simulink model "Receiver"  (R2017b)
settings: Solver=FixedStepDiscrete  StartTime=0.0  StopTime=10.0  RelTol=1e-3
InitFcn:
  | modelSettings
undefined symbols (not defined in the file or in its folder): crcDecodeLag, numTrainingSamples, RadioSampleRate, VibertiTracebackLength, xPreambleSeq
libraries: dsphdlfiltering x19, simulink x7, hdlsllib x4, commdigbbndpm3 x2, commcrc2 x1, dspstat3 x1, commseqgen3 x1, commutil2 x1, commcnvcod2 x1
(part 1 of 2)
settings Model: DataTypeOverride=Off  MinMaxOverflowLogging=MinMaxAndOverflow  FPTRunName=NoOverride  Creator=tcollins  LastModifiedBy=tcollins
settings DataIOCC: SaveOutput=off  SaveTime=off
settings OptimizationCC: BlockReduction=off  ConditionallyExecuteInputs=off  DefaultParameterBehavior=Inlined
settings DebuggingCC: AlgebraicLoopMsg=error  SingleTaskRateTransMsg=error
settings HardwareCC: ProdBitPerPointer=32  ProdBitPerSizeT=32  ProdBitPerPtrDiffT=32  ProdLargestAtomicFloat=None  ProdIntDivRoundTo=Undefined  ProdEndianess=Unspecified  ProdWordSize=32  ProdHWDeviceType=ASIC/FPGA->ASIC/FPGA  ProdEqTarget=off
settings CodeAppCC: StateflowObjectComments=on
settings SimscapeCC: SimscapeNormalizeSystem=off

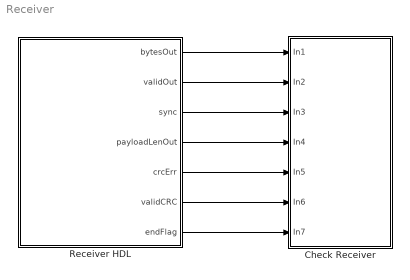
== system Receiver ==
  Check Receiver : Subsystem
  Receiver HDL : Subsystem  TreatAsAtomicUnit=on
      mask Display:
      | if ispc
      |     d = '\';
      | else
      |     d = '/';
      | end
      | model_path = get_param(bdroot, 'FileName');
      | %info = Simulink.MDLInfo(bdroot)
      | c = strsplit(model_path,d); c = strjoin(c(1:end-2),d);
      | logo = [c,d,'ADI_logo.svg'];
      | %disp(logo);
      | image(logo);
  wires:
  Receiver HDL/1(bytesOut) -> Check Receiver/1(In1)
  Receiver HDL/2(validOut) -> Check Receiver/2(In2)
  Receiver HDL/3(sync) -> Check Receiver/3(In3)
  Receiver HDL/4(payloadLenOut) -> Check Receiver/4(In4)
  Receiver HDL/5(crcErr) -> Check Receiver/5(In5)
  Receiver HDL/6(validCRC) -> Check Receiver/6(In6)
  Receiver HDL/7(endFlag) -> Check Receiver/7(In7)

== system Receiver/Check Receiver ==
  In1 : Inport
  In2 : Inport  Port=2
  In3 : Inport  Port=3
  In4 : Inport  Port=4
  In5 : Inport  Port=5
  In6 : Inport  Port=6
  In7 : Inport  Port=7
  DMA Capture : MATLAB Function  TreatAsAtomicUnit=on
  Terminator : Terminator
  Terminator1 : Terminator
  Terminator2 : Terminator
  wires:
  In3/1 -> DMA Capture/3(sync)
  In2/1 -> DMA Capture/2(validOut)
  In1/1 -> DMA Capture/1(bytes)
  In4/1 -> DMA Capture/4(payloadLen)
  In7/1 -> Terminator/1
  In5/1 -> Terminator1/1
  In6/1 -> Terminator2/1

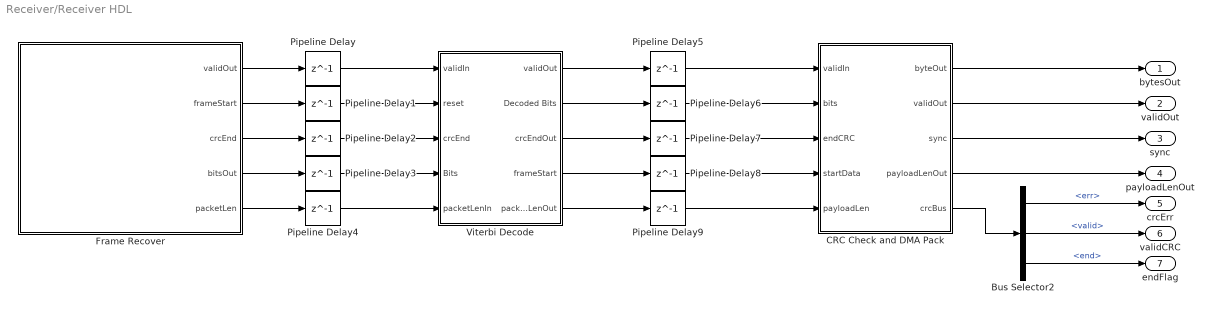
== system Receiver/Receiver HDL ==
  Bus Selector2 : BusSelector  OutputSignals=err,valid,end
  CRC Check and DMA Pack : Subsystem
  Frame Recover : Subsystem
  Pipeline Delay{,1..9} (10 alike) : Delay  DelayLength=1
  Viterbi Decode : Subsystem  TreatAsAtomicUnit=on
  bytesOut : Outport
  validOut : Outport  Port=2
  sync : Outport  Port=3
  payloadLenOut : Outport  Port=4
  crcErr : Outport  Port=5
  validCRC : Outport  Port=6
  endFlag : Outport  Port=7
  wires:
  Bus Selector2/3 -> endFlag/1  "<end>"
  Bus Selector2/2 -> validCRC/1  "<valid>"
  Bus Selector2/1 -> crcErr/1  "<err>"
  CRC Check and DMA Pack/5(crcBus) -> Bus Selector2/1
  Frame Recover/5(packetLen) -> Pipeline Delay4/1
  Frame Recover/1(validOut) -> Pipeline Delay/1
  Frame Recover/2(frameStart) -> Pipeline Delay1/1
  Frame Recover/3(crcEnd) -> Pipeline Delay2/1
  Frame Recover/4(bitsOut) -> Pipeline Delay3/1
  Viterbi Decode/3(crcEndOut) -> Pipeline Delay7/1
  Viterbi Decode/4(frameStart) -> Pipeline Delay8/1
  Viterbi Decode/5(packetLenOut) -> Pipeline Delay9/1
  CRC Check and DMA Pack/1(byteOut) -> bytesOut/1
  CRC Check and DMA Pack/2(validOut) -> validOut/1
  Pipeline Delay1/1 -> Viterbi Decode/2(reset)
  Pipeline Delay3/1 -> Viterbi Decode/4(Bits)
  Pipeline Delay4/1 -> Viterbi Decode/5(packetLenIn)
  Pipeline Delay8/1 -> CRC Check and DMA Pack/4(startData)
  Pipeline Delay6/1 -> CRC Check and DMA Pack/2(bits)
  Pipeline Delay9/1 -> CRC Check and DMA Pack/5(payloadLen)
  Pipeline Delay7/1 -> CRC Check and DMA Pack/3(endCRC)
  CRC Check and DMA Pack/3(sync) -> sync/1
  Pipeline Delay2/1 -> Viterbi Decode/3(crcEnd)
  Viterbi Decode/2(Decoded Bits) -> Pipeline Delay6/1
  CRC Check and DMA Pack/4(payloadLenOut) -> payloadLenOut/1
  Pipeline Delay/1 -> Viterbi Decode/1(validIn)
  Viterbi Decode/1(validOut) -> Pipeline Delay5/1
  Pipeline Delay5/1 -> CRC Check and DMA Pack/1(validIn)

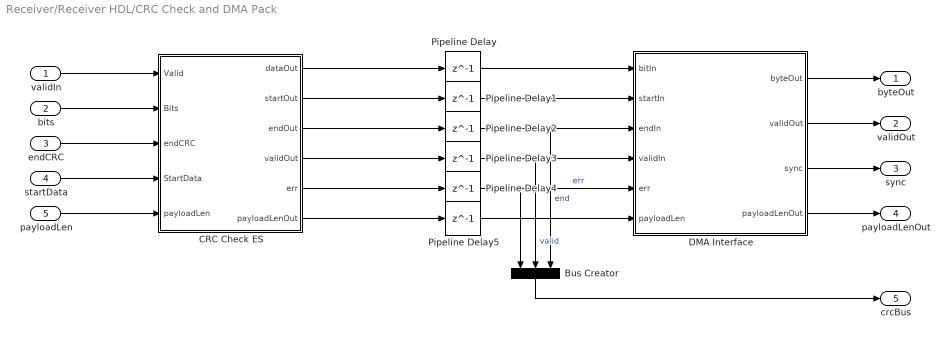
== system Receiver/Receiver HDL/CRC Check and DMA Pack ==
  validIn : Inport
  bits : Inport  Port=2
  endCRC : Inport  Port=3
  startData : Inport  Port=4
  payloadLen : Inport  Port=5
  Bus Creator : BusCreator  Inputs=3
  CRC Check ES : Subsystem
  DMA Interface : Subsystem
  Pipeline Delay{,1..5} (6 alike) : Delay  DelayLength=1
  byteOut : Outport
  validOut : Outport  Port=2
  sync : Outport  Port=3
  payloadLenOut : Outport  Port=4
  crcBus : Outport  Port=5
  wires:
  Bus Creator/1 -> crcBus/1
  DMA Interface/2(validOut) -> validOut/1
  CRC Check ES/3(endOut) -> Pipeline Delay2/1
  DMA Interface/1(byteOut) -> byteOut/1
  CRC Check ES/2(startOut) -> Pipeline Delay1/1
  CRC Check ES/1(dataOut) -> Pipeline Delay/1
  CRC Check ES/5(err) -> Pipeline Delay4/1
  bits/1 -> CRC Check ES/2(Bits)
  DMA Interface/3(sync) -> sync/1
  payloadLen/1 -> CRC Check ES/5(payloadLen)
  startData/1 -> CRC Check ES/4(StartData)
  CRC Check ES/6(payloadLenOut) -> Pipeline Delay5/1
  endCRC/1 -> CRC Check ES/3(endCRC)
  Pipeline Delay/1 -> DMA Interface/1(bitIn)
  Pipeline Delay1/1 -> DMA Interface/2(startIn)
  Pipeline Delay2/1 -> DMA Interface/3(endIn), Bus Creator/3  "end"
  Pipeline Delay3/1 -> DMA Interface/4(validIn), Bus Creator/2  "valid"
  Pipeline Delay4/1 -> DMA Interface/5(err), Bus Creator/1  "err"
  Pipeline Delay5/1 -> DMA Interface/6(payloadLen)
  validIn/1 -> CRC Check ES/1(Valid)
  DMA Interface/4(payloadLenOut) -> payloadLenOut/1
  CRC Check ES/4(validOut) -> Pipeline Delay3/1

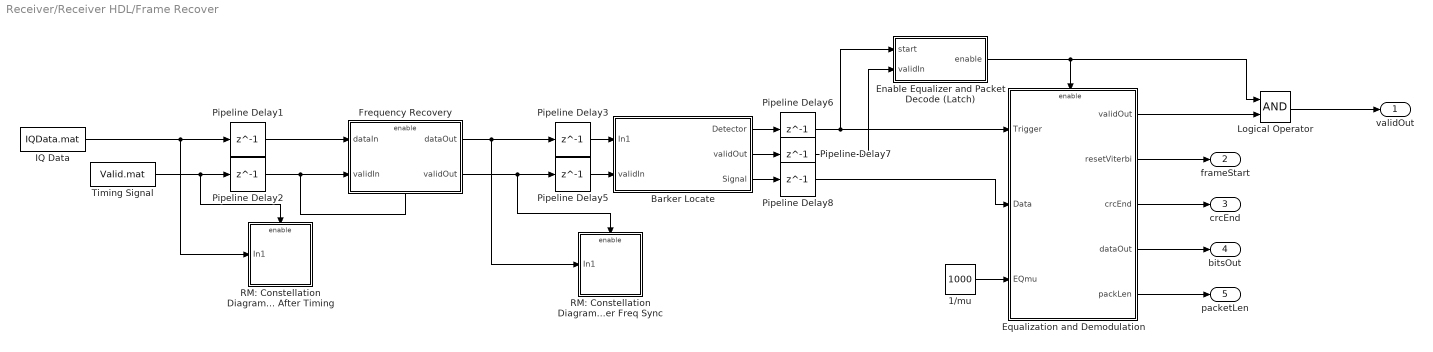
== system Receiver/Receiver HDL/Frame Recover ==
  1/mu : Constant  Value=1000  OutDataTypeStr=int16  SampleTime=-1
  Barker Locate : Subsystem  mask{Threshold=1}
  Enable Equalizer and Packet Decode (Latch) : MATLAB Function  TreatAsAtomicUnit=on
  Equalization and Demodulation : Subsystem
  Frequency Recovery : Subsystem
  IQ Data : FromFile  FileName=IQData.mat  SampleTime=1/RadioSampleRate
  Logical Operator : Logic  AllPortsSameDT=off  OutDataTypeStr=boolean
  Pipeline Delay{1..3,5..8} (7 alike) : Delay  DelayLength=1
  RM: Constellation Diagram After Freq Sync : Subsystem
  RM: Constellation Diagram After Timing : Subsystem
  Timing Signal : FromFile  FileName=Valid.mat  SampleTime=1/RadioSampleRate
  validOut : Outport
  frameStart : Outport  Port=2
  crcEnd : Outport  Port=3
  bitsOut : Outport  Port=4
  packetLen : Outport  Port=5
  wires:
  Equalization and Demodulation/2(resetViterbi) -> frameStart/1
  Barker Locate/2(validOut) -> Pipeline Delay7/1
  Equalization and Demodulation/3(crcEnd) -> crcEnd/1
  Enable Equalizer and Packet Decode (Latch)/1(enable) -> Logical Operator/1, Equalization and Demodulation/Enable
  Equalization and Demodulation/4(dataOut) -> bitsOut/1
  Barker Locate/3(Signal) -> Pipeline Delay8/1
  Equalization and Demodulation/1(validOut) -> Logical Operator/2
  Equalization and Demodulation/5(packLen) -> packetLen/1
  Barker Locate/1(Detector) -> Pipeline Delay6/1
  Pipeline Delay1/1 -> Frequency Recovery/1(dataIn)
  Pipeline Delay2/1 -> Frequency Recovery/Enable, Frequency Recovery/2(validIn)
  Pipeline Delay3/1 -> Barker Locate/1(In1)
  Pipeline Delay5/1 -> Barker Locate/2(validIn)
  Pipeline Delay6/1 -> Enable Equalizer and Packet Decode (Latch)/1(start), Equalization and Demodulation/1(Trigger)
  Pipeline Delay7/1 -> Enable Equalizer and Packet Decode (Latch)/2(validIn)
  Pipeline Delay8/1 -> Equalization and Demodulation/2(Data)
  Logical Operator/1 -> validOut/1
  Timing Signal/1 -> Pipeline Delay2/1, RM: Constellation Diagram After Timing/Enable
  IQ Data/1 -> RM: Constellation Diagram After Timing/1(In1), Pipeline Delay1/1
  1/mu/1 -> Equalization and Demodulation/3(EQmu)
  Frequency Recovery/1(dataOut) -> Pipeline Delay3/1, RM: Constellation Diagram After Freq Sync/1(In1)
  Frequency Recovery/2(validOut) -> RM: Constellation Diagram After Freq Sync/Enable, Pipeline Delay5/1

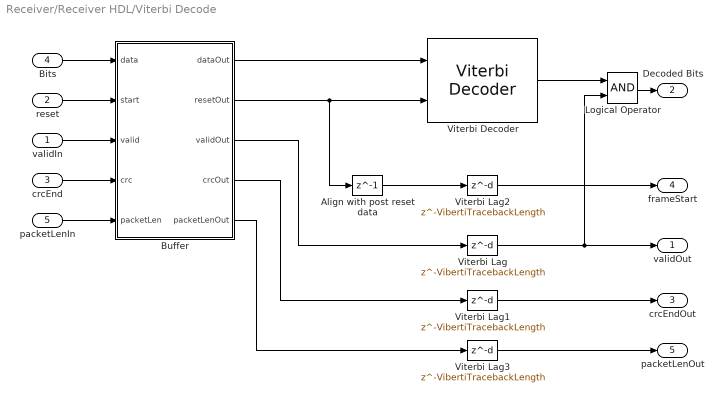
== system Receiver/Receiver HDL/Viterbi Decode ==
  validIn : Inport
  reset : Inport  Port=2
  crcEnd : Inport  Port=3
  Bits : Inport  Port=4
  packetLenIn : Inport  Port=5
  Align with post reset data : Delay  DelayLength=1
  Buffer : Subsystem
  Logical Operator : Logic  AllPortsSameDT=off  OutDataTypeStr=boolean
  Viterbi Decoder : commcnvcod2/Viterbi Decoder  trellis=poly2trellis(7, [171 133])  isPunctured=off  punctureVector=[1; 1; 0; 1; 0; 1]  erasures=off  dectype=Hard decision  nsdecb=4  runSigValErrCheck=off  tbdepth=VibertiTracebackLength  opmode=Continuous  reset=on  delayedResetAction=on  smWordLength=16  outDataType=boolean
      settings: SourceProductName=Communications System Toolbox  SourceProductBaseCode=CM
  Viterbi Lag{,1..3} (4 alike) : Delay  DelayLength=VibertiTracebackLength
  validOut : Outport  InitialOutput=0
  Decoded Bits : Outport  Port=2  InitialOutput=0
  crcEndOut : Outport  Port=3  InitialOutput=0
  frameStart : Outport  Port=4  InitialOutput=0
  packetLenOut : Outport  Port=5  InitialOutput=0
  wires:
  Viterbi Lag3/1 -> packetLenOut/1
  packetLenIn/1 -> Buffer/5(packetLen)
  Viterbi Lag2/1 -> frameStart/1
  Bits/1 -> Buffer/1(data)
  reset/1 -> Buffer/2(start)
  validIn/1 -> Buffer/3(valid)
  crcEnd/1 -> Buffer/4(crc)
  Buffer/1(dataOut) -> Viterbi Decoder/1
  Buffer/2(resetOut) -> Align with post reset data/1, Viterbi Decoder/2
  Buffer/3(validOut) -> Viterbi Lag/1
  Viterbi Lag1/1 -> crcEndOut/1
  Viterbi Lag/1 -> Logical Operator/2, validOut/1
  Buffer/5(packetLenOut) -> Viterbi Lag3/1
  Align with post reset data/1 -> Viterbi Lag2/1
  Logical Operator/1 -> Decoded Bits/1
  Viterbi Decoder/1 -> Logical Operator/1
  Buffer/4(crcOut) -> Viterbi Lag1/1

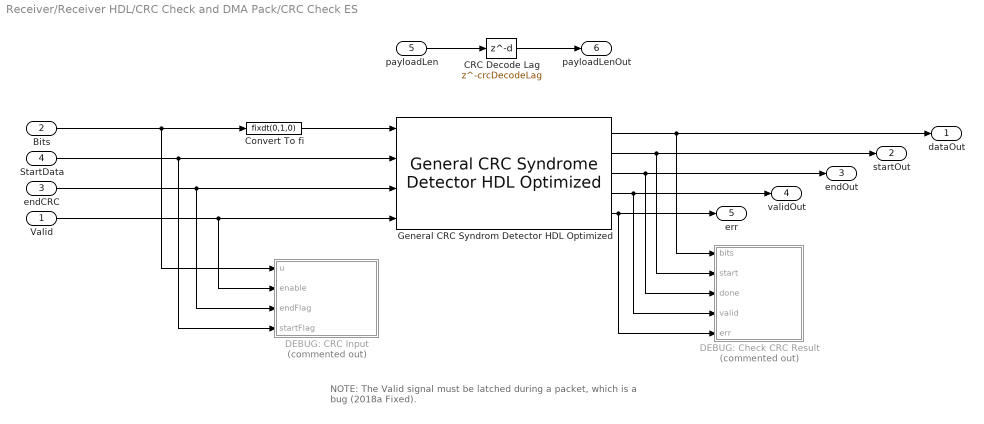
== system Receiver/Receiver HDL/CRC Check and DMA Pack/CRC Check ES ==
  note: NOTE:
      | 	The Valid signal must be latched during a packet, which is
      | 	a bug (2018a Fixed).
  Valid : Inport
  Bits : Inport  Port=2
  endCRC : Inport  Port=3
  StartData : Inport  Port=4
  payloadLen : Inport  Port=5
  CRC Decode Lag : Delay  DelayLength=crcDecodeLag
  Convert To fi : DataTypeConversion  OutDataTypeStr=fixdt(0,1,0)  SaturateOnIntegerOverflow=on
  DEBUG: CRC Input : MATLAB Function  Commented=on  TreatAsAtomicUnit=on
  DEBUG: Check CRC Result : MATLAB Function  Commented=on  TreatAsAtomicUnit=on
  General CRC Syndrom Detector HDL Optimized : commcrc2/General CRC Syndrome Detector HDL Optimized  Polynomial=crc32Poly  InitialState=0  DirectMethod=off  ReflectInput=off  ReflectCRCChecksum=off  FinalXORValue=0  SimulateUsing=Code generation
      settings: SourceProductName=Communications System Toolbox  SourceProductBaseCode=CM
  dataOut : Outport  InitialOutput=0
  startOut : Outport  Port=2  InitialOutput=0
  endOut : Outport  Port=3  InitialOutput=0
  validOut : Outport  Port=4  InitialOutput=0
  err : Outport  Port=5  InitialOutput=0
  payloadLenOut : Outport  Port=6  InitialOutput=0
  wires:
  Bits/1 -> Convert To fi/1, DEBUG: CRC Input/1(u)
  General CRC Syndrom Detector HDL Optimized/1 -> DEBUG: Check CRC Result/1(bits), dataOut/1
  General CRC Syndrom Detector HDL Optimized/3 -> DEBUG: Check CRC Result/3(done), endOut/1
  General CRC Syndrom Detector HDL Optimized/4 -> DEBUG: Check CRC Result/4(valid), validOut/1
  General CRC Syndrom Detector HDL Optimized/5 -> DEBUG: Check CRC Result/5(err), err/1
  General CRC Syndrom Detector HDL Optimized/2 -> DEBUG: Check CRC Result/2(start), startOut/1
  Convert To fi/1 -> General CRC Syndrom Detector HDL Optimized/1
  payloadLen/1 -> CRC Decode Lag/1
  CRC Decode Lag/1 -> payloadLenOut/1
  StartData/1 -> DEBUG: CRC Input/4(startFlag), General CRC Syndrom Detector HDL Optimized/2
  endCRC/1 -> DEBUG: CRC Input/3(endFlag), General CRC Syndrom Detector HDL Optimized/3
  Valid/1 -> General CRC Syndrom Detector HDL Optimized/4, DEBUG: CRC Input/2(enable)

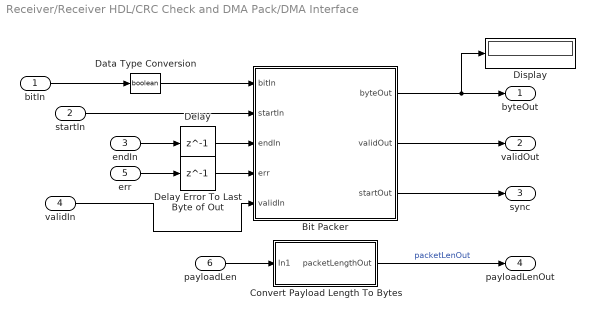
== system Receiver/Receiver HDL/CRC Check and DMA Pack/DMA Interface ==
  bitIn : Inport
  startIn : Inport  Port=2
  endIn : Inport  Port=3
  validIn : Inport  Port=4
  err : Inport  Port=5
  payloadLen : Inport  Port=6
  Bit Packer : MATLAB Function  TreatAsAtomicUnit=on
  Convert Payload Length To Bytes : Subsystem
  Data Type Conversion : DataTypeConversion  OutDataTypeStr=boolean
  Delay : Delay  DelayLength=1
  Delay Error To Last Byte of Out : Delay  DelayLength=1
  Display : Display
  byteOut : Outport
  validOut : Outport  Port=2
  sync : Outport  Port=3
  payloadLenOut : Outport  Port=4
  wires:
  bitIn/1 -> Data Type Conversion/1
  Delay/1 -> Bit Packer/3(endIn)
  Delay Error To Last Byte of Out/1 -> Bit Packer/4(err)
  Bit Packer/2(validOut) -> validOut/1
  Bit Packer/3(startOut) -> sync/1
  Bit Packer/1(byteOut) -> Display/1, byteOut/1
  err/1 -> Delay Error To Last Byte of Out/1
  validIn/1 -> Bit Packer/5(validIn)
  endIn/1 -> Delay/1
  startIn/1 -> Bit Packer/2(startIn)
  Data Type Conversion/1 -> Bit Packer/1(bitIn)
  payloadLen/1 -> Convert Payload Length To Bytes/1(In1)
  Convert Payload Length To Bytes/1(packetLengthOut) -> payloadLenOut/1  "packetLenOut"

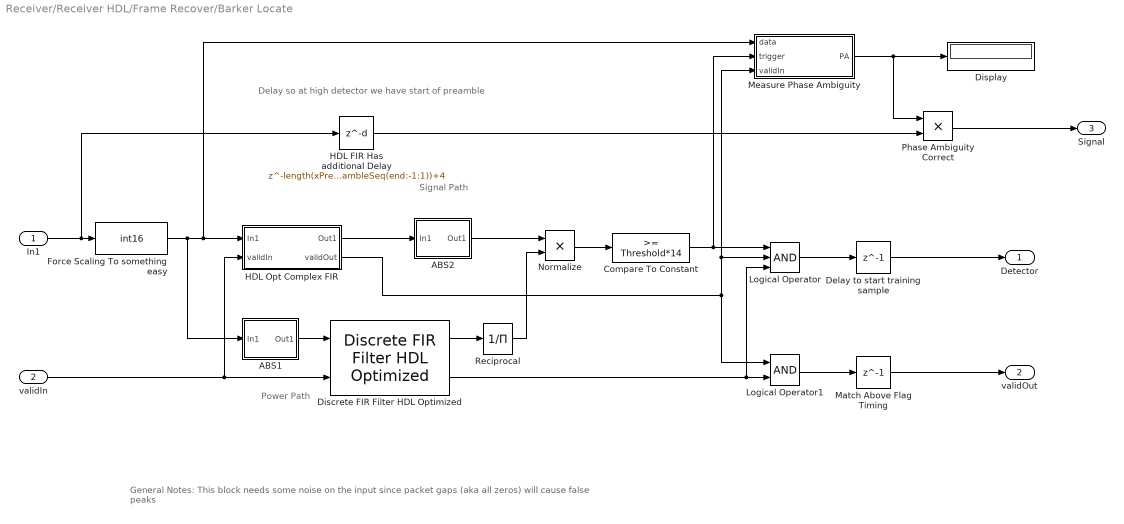
== system Receiver/Receiver HDL/Frame Recover/Barker Locate ==
  note: General Notes:
      | This block needs some noise on the input since packet gaps (aka all zeros) will cause false peaks
  note: Delay so at high detector we have start of preamble
  note: Power Path
  note: Signal Path
  In1 : Inport  PortDimensions=1
  validIn : Inport  Port=2  PortDimensions=1
  ABS1 : Subsystem
  ABS2 : Subsystem
  Compare To Constant : simulink/Logic and Bit Operations/Compare To Constant  relop=>=  const=Threshold*14  OutDataTypeStr=boolean
  "Delay to start training sample " : Delay  DelayLength=1
  Discrete FIR Filter HDL Optimized : dsphdlfiltering/Discrete FIR Filter HDL Optimized  Numerator=ones(1,length(xPreambleSeq)*1)/1  Sharing=off  SharingFactor=2  SimulateUsing=Code generation  roundingMode=Floor  overflowMode=off  CoefficientsDataTypeStr=Inherit: Same word length as input  CoefficientsMin=[]  CoefficientsMax=[]  OutputDataTypeStr=fixdt(1,17,0)  OutputMin=[]  OutputMax=[]  ValidInPort=on  ReadyPort=off
      settings: SourceProductName=DSP System Toolbox  SourceProductBaseCode=DS
  Display : Display
  Force Scaling To something easy : DataTypeConversion  OutDataTypeStr=int16  SaturateOnIntegerOverflow=on
  HDL FIR Has additional Delay : Delay  DelayLength=length(xPreambleSeq(end:-1:1))+4
  HDL Opt Complex FIR : Subsystem  mask{Taps=xPreambleSeq(end:-1:1).'}
  Logical Operator : Logic  Inputs=3  AllPortsSameDT=off  OutDataTypeStr=boolean
  Logical Operator1 : Logic  AllPortsSameDT=off  OutDataTypeStr=boolean
  Match Above Flag Timing : Delay  DelayLength=1
  Measure Phase Ambiguity : Subsystem
  Normalize : Product  Inputs=**  OutDataTypeStr=int16  RndMeth=Simplest  SaturateOnIntegerOverflow=on
  Phase Ambiguity Correct : Product  OutDataTypeStr=fixdt(1,16,14)
  Reciprocal : Product  Inputs=/  SaturateOnIntegerOverflow=on  RndMeth=Zero
  Detector : Outport
  validOut : Outport  Port=2
  Signal : Outport  Port=3
  wires:
  HDL Opt Complex FIR/1(Out1) -> ABS2/1(In1)
  ABS2/1(Out1) -> Normalize/1
  "Delay to start training sample "/1 -> Detector/1
  Normalize/1 -> Compare To Constant/1
  In1/1 -> HDL FIR Has additional Delay/1, Force Scaling To something easy/1
  ABS1/1(Out1) -> Discrete FIR Filter HDL Optimized/1
  Logical Operator/1 -> "Delay to start training sample "/1
  Logical Operator1/1 -> Match Above Flag Timing/1
  Measure Phase Ambiguity/1(PA) -> Display/1, Phase Ambiguity Correct/1
  validIn/1 -> HDL Opt Complex FIR/2(validIn), Discrete FIR Filter HDL Optimized/2
  Discrete FIR Filter HDL Optimized/2 -> Logical Operator1/2, Logical Operator/3
  HDL Opt Complex FIR/2(validOut) -> Logical Operator1/1, Measure Phase Ambiguity/3(validIn), Logical Operator/2
  Phase Ambiguity Correct/1 -> Signal/1
  HDL FIR Has additional Delay/1 -> Phase Ambiguity Correct/2
  Force Scaling To something easy/1 -> ABS1/1(In1), HDL Opt Complex FIR/1(In1), Measure Phase Ambiguity/1(data)
  Compare To Constant/1 -> Measure Phase Ambiguity/2(trigger), Logical Operator/1
  Discrete FIR Filter HDL Optimized/1 -> Reciprocal/1
  Reciprocal/1 -> Normalize/2
  Match Above Flag Timing/1 -> validOut/1

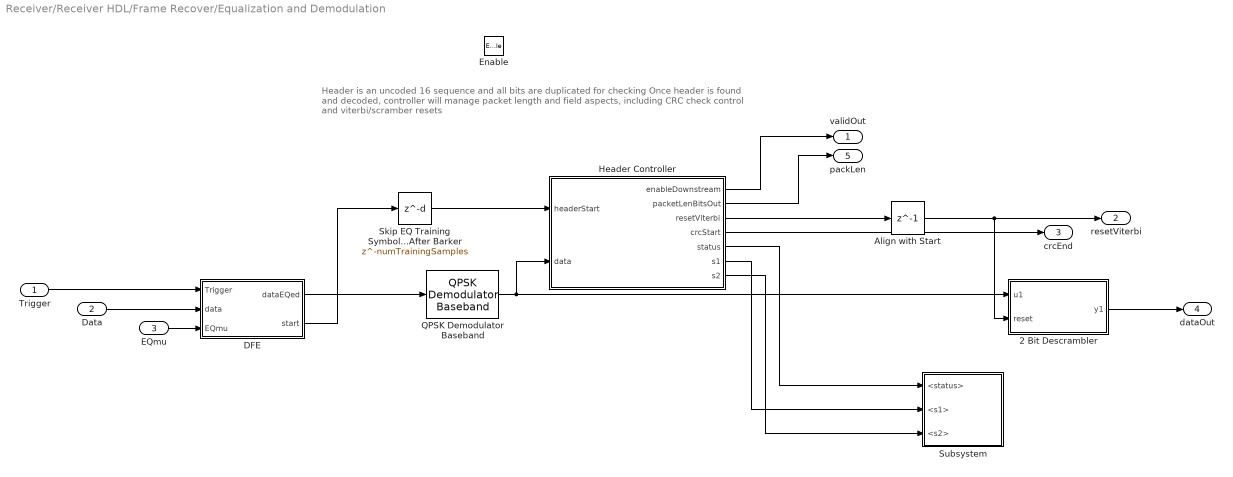
== system Receiver/Receiver HDL/Frame Recover/Equalization and Demodulation ==
  note: Header is an uncoded 16 sequence and all bits are duplicated for checking
      |
      | Once header is found and decoded, controller will manage packet length and field aspects,
      | including CRC check control and viterbi/scramber resets
  Trigger : Inport
  Data : Inport  Port=2
  EQmu : Inport  Port=3
  Enable : EnablePort
  2 Bit Descrambler : Subsystem  mask{polynom=[1 1 0 1 0 1 0 1], initstate=[0 1 0 0 0 1 0]}
      mask prompts: polynom "Polynomial"; initstate "Inital State"
      mask Display: fprintf('HDL Descrambler')
  Align with Start : Delay  DelayLength=1
  DFE : Subsystem
  Header Controller : MATLAB Function  TreatAsAtomicUnit=on
  QPSK Demodulator Baseband : commdigbbndpm3/QPSK Demodulator Baseband  OutType=Bit  DecType=Hard decision  VarSource=Dialog  Variance=1  Dec=Binary  Ph=pi/4  outDtype1=boolean  outDtype2=Inherit via internal rule  derotateFactorWordLen=16  derotateFactorDataTypeStr=Inherit: Same word length as input  derotateFactorLastDataTypeStr=Inherit: Same word length as input
  Skip EQ Training Symbols After Barker : Delay  DelayLength=numTrainingSamples
  Subsystem : Subsystem
  validOut : Outport  InitialOutput=0
  resetViterbi : Outport  Port=2  InitialOutput=0
  crcEnd : Outport  Port=3  InitialOutput=0
  dataOut : Outport  Port=4  InitialOutput=0
  packLen : Outport  Port=5  InitialOutput=0
  wires:
  Skip EQ Training Symbols After Barker/1 -> Header Controller/1(headerStart)
  DFE/1(dataEQed) -> QPSK Demodulator Baseband/1
  Header Controller/2(packetLenBitsOut) -> packLen/1
  Header Controller/3(resetViterbi) -> Align with Start/1
  Header Controller/4(crcStart) -> crcEnd/1
  QPSK Demodulator Baseband/1 -> 2 Bit Descrambler/1(u1), Header Controller/2(data)
  2 Bit Descrambler/1(y1) -> dataOut/1
  Trigger/1 -> DFE/1(Trigger)
  Data/1 -> DFE/2(data)
  DFE/2(start) -> Skip EQ Training Symbols After Barker/1
  EQmu/1 -> DFE/3(EQmu)
  Header Controller/5(status) -> Subsystem/1(<status>)
  Header Controller/6(s1) -> Subsystem/2(<s1>)
  Header Controller/7(s2) -> Subsystem/3(<s2>)
  Align with Start/1 -> 2 Bit Descrambler/2(reset), resetViterbi/1
  Header Controller/1(enableDownstream) -> validOut/1

== system Receiver/Receiver HDL/Frame Recover/Frequency Recovery ==
  dataIn : Inport
  validIn : Inport  Port=2
  Enable : EnablePort
  Complex Phase Shift : commutil2/Complex Phase Shift
      settings: SourceProductName=Communications System Toolbox  SourceProductBaseCode=CM
  Data Type Conversion : DataTypeConversion  OutDataTypeStr=fixdt(1,16,13)
  Data Type Conversion1 : DataTypeConversion  OutDataTypeStr=double
  Delay : Delay  DelayLength=1
  Loop Filter : Subsystem  mask{BnTs=0.1, zeta=3*1/sqrt(2), N=1}
      mask prompts: BnTs "Normalized Loop Bandwidth"; zeta "Damping Factor"; N "Number of Samples/Symbol"
      mask init:
      | % See C.57 to C.61 in Michael Rice's "Digital Communications 
      | % - A Discrete-Time Approach" for details
      | 
      | %theta = BnTs/(zeta+0.25/zeta);  %0.0385
      | %d = 1 + 2*zeta*theta + theta*theta; %1.1938
      | %K1 = zeta*theta/d; %0.0805
      | %K2 = theta*theta/(d*2); %6.1958e-04
      | 
      | %%
      | DampingFactor = zeta;
      | samplesPerSymbol = N;
      | NormalizedLoopBandwidth = BnTs;
      | %
      | PhaseRecoveryLoopBandwidth = NormalizedLoopBandwidth*samplesPerSymbol;
      |  
      | PhaseRecoveryGain = samplesPerSymbol;
      |  
      | PhaseErrorDetectorGain = 1;
      | 
      | 
      | theta = PhaseRecoveryLoopBandwidth/...
      |     ((DampingFactor + 0.25/DampingFactor)*samplesPerSymbol);
      |  
      | d = 1 + 2*DampingFactor*theta + theta*theta;
      |  
      | % K1
      | K1 = (4*DampingFactor*theta/d)/...
      |     (PhaseErrorDetectorGain*PhaseRecoveryGain);
      | % K2
      | K2 = (4/samplesPerSymbol*theta*theta/d)/...
      |     (PhaseErrorDetectorGain*PhaseRecoveryGain);
      mask Display: disp('Loop Filter')
  PED : MATLAB Function  TreatAsAtomicUnit=on
  Phase Error : Scope
  State Control : StateControl  StateControl=Synchronous
  dataOut : Outport
  validOut : Outport  Port=2
  wires:
  validIn/1 -> validOut/1
  Complex Phase Shift/1 -> Delay/1
  dataIn/1 -> Data Type Conversion1/1
  Loop Filter/1(v) -> Complex Phase Shift/2
  PED/1(e) -> Loop Filter/1(e), Phase Error/1
  Delay/1 -> PED/1(In), Data Type Conversion/1
  Data Type Conversion1/1 -> Complex Phase Shift/1
  Data Type Conversion/1 -> dataOut/1

== system Receiver/Receiver HDL/Frame Recover/RM: Constellation Diagram After Freq Sync ==
  In1 : Inport
  Enable : EnablePort
  After Frequency Recovery : ConstellationDiagram
  wires:
  In1/1 -> After Frequency Recovery/1

== system Receiver/Receiver HDL/Frame Recover/RM: Constellation Diagram After Timing ==
  In1 : Inport
  Enable : EnablePort
  After Timing Recovery : ConstellationDiagram
  wires:
  In1/1 -> After Timing Recovery/1

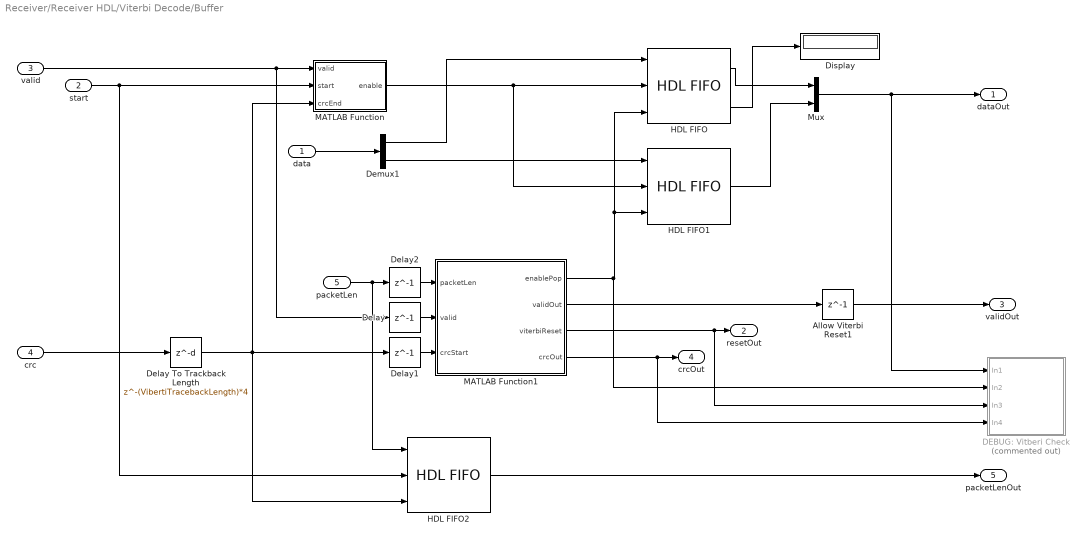
== system Receiver/Receiver HDL/Viterbi Decode/Buffer ==
  data : Inport
  start : Inport  Port=2
  valid : Inport  Port=3
  crc : Inport  Port=4
  packetLen : Inport  Port=5
  Allow Viterbi Reset1 : Delay  DelayLength=1
  DEBUG: Vitberi Check : Subsystem  Commented=on
  Delay : Delay  DelayLength=1
  Delay To Trackback Length : Delay  DelayLength=(VibertiTracebackLength)*4
  Delay1 : Delay  DelayLength=1
  Delay2 : Delay  DelayLength=1
  Demux1 : Demux  Outputs=2
  Display : Display
  HDL FIFO : hdlsllib/HDL RAMs/HDL FIFO  fifo_size=2^16  ratio=1  push_msg=Warning  pop_msg=Warning  show_empty=off  show_full=off  show_num=on
      settings: SourceProductName=HDL Coder  SourceProductBaseCode=HD
  HDL FIFO1 : hdlsllib/HDL RAMs/HDL FIFO  fifo_size=2^16  ratio=1  push_msg=Warning  pop_msg=Warning  show_empty=off  show_full=off  show_num=off
      settings: SourceProductName=HDL Coder  SourceProductBaseCode=HD
  HDL FIFO2 : hdlsllib/HDL RAMs/HDL FIFO  fifo_size=2^3  ratio=1  push_msg=Warning  pop_msg=Warning  show_empty=off  show_full=off  show_num=off
      settings: SourceProductName=HDL Coder  SourceProductBaseCode=HD
  MATLAB Function : MATLAB Function  TreatAsAtomicUnit=on
  MATLAB Function1 : MATLAB Function  TreatAsAtomicUnit=on
  Mux : Mux  Inputs=2
  dataOut : Outport
  resetOut : Outport  Port=2
  validOut : Outport  Port=3
  crcOut : Outport  Port=4  OutDataTypeStr=boolean
  packetLenOut : Outport  Port=5
  wires:
  Demux1/1 -> HDL FIFO/1
  data/1 -> Demux1/1
  HDL FIFO/1 -> Mux/1
  HDL FIFO1/1 -> Mux/2
  Demux1/2 -> HDL FIFO1/1
  MATLAB Function/1(enable) -> HDL FIFO1/2, HDL FIFO/2
  HDL FIFO/2 -> Display/1
  HDL FIFO2/1 -> packetLenOut/1
  packetLen/1 -> Delay2/1, HDL FIFO2/1
  valid/1 -> Delay/1, MATLAB Function/1(valid)
  start/1 -> MATLAB Function/2(start), HDL FIFO2/2
  Delay/1 -> MATLAB Function1/2(valid)
  Delay1/1 -> MATLAB Function1/3(crcStart)
  Delay2/1 -> MATLAB Function1/1(packetLen)
  MATLAB Function1/1(enablePop) -> DEBUG: Vitberi Check/2(In2), HDL FIFO1/3, HDL FIFO/3
  Allow Viterbi Reset1/1 -> validOut/1
  crc/1 -> Delay To Trackback Length/1
  Mux/1 -> DEBUG: Vitberi Check/1(In1), dataOut/1
  Delay To Trackback Length/1 -> Delay1/1, MATLAB Function/3(crcEnd), HDL FIFO2/3
  MATLAB Function1/2(validOut) -> Allow Viterbi Reset1/1
  MATLAB Function1/4(crcOut) -> DEBUG: Vitberi Check/4(In4), crcOut/1
  MATLAB Function1/3(viterbiReset) -> DEBUG: Vitberi Check/3(In3), resetOut/1

== system Receiver/Receiver HDL/CRC Check and DMA Pack/DMA Interface/Convert Payload Length To Bytes ==
  In1 : Inport
  Constant : Constant  Value=uint16(32-1)  SampleTime=-1
  Convert To Bytes From Bits : ArithShift  BitShiftNumber=3  BitShiftDirection=Right
  Convert To Uncoded : ArithShift  BitShiftNumber=1  BitShiftDirection=Right
  Data Type Conversion : DataTypeConversion  OutDataTypeStr=uint16
  Remove CRC Length : Sum  Inputs=+-  AccumDataTypeStr=uint16
  packetLengthOut : Outport
  wires:
  In1/1 -> Convert To Uncoded/1
  Remove CRC Length/1 -> Convert To Bytes From Bits/1
  Convert To Uncoded/1 -> Remove CRC Length/1
  Convert To Bytes From Bits/1 -> Data Type Conversion/1
  Constant/1 -> Remove CRC Length/2
  Data Type Conversion/1 -> packetLengthOut/1

== system Receiver/Receiver HDL/Frame Recover/Barker Locate/ABS1 ==
  In1 : Inport
  Add : Sum
  Complex to Real-Imag : ComplexToRealImag
  Product : Product  OutDataTypeStr=int16
  Product1 : Product  OutDataTypeStr=int16
  Out1 : Outport
  wires:
  In1/1 -> Complex to Real-Imag/1
  Complex to Real-Imag/2 -> Product1/2, Product1/1
  Complex to Real-Imag/1 -> Product/1, Product/2
  Product/1 -> Add/1
  Product1/1 -> Add/2
  Add/1 -> Out1/1

== system Receiver/Receiver HDL/Frame Recover/Barker Locate/ABS2 ==
  In1 : Inport
  Add : Sum  SaturateOnIntegerOverflow=on
  Complex to Real-Imag : ComplexToRealImag
  Product : Product  OutDataTypeStr=int16
  Product1 : Product  OutDataTypeStr=int16
  Out1 : Outport
  wires:
  In1/1 -> Complex to Real-Imag/1
  Complex to Real-Imag/2 -> Product1/2, Product1/1
  Complex to Real-Imag/1 -> Product/1, Product/2
  Product/1 -> Add/1
  Product1/1 -> Add/2
  Add/1 -> Out1/1

== system Receiver/Receiver HDL/Frame Recover/Barker Locate/HDL Opt Complex FIR ==
  In1 : Inport
  validIn : Inport  Port=2
  Add : Sum  AccumDataTypeStr=fixdt(1,16,0)
  Discrete FIR Filter HDL Optimized : dsphdlfiltering/Discrete FIR Filter HDL Optimized  Numerator=real(Taps)  Sharing=off  SharingFactor=2  SimulateUsing=Code generation  roundingMode=Floor  overflowMode=off  CoefficientsDataTypeStr=Inherit: Same word length as input  CoefficientsMin=[]  CoefficientsMax=[]  OutputDataTypeStr=fixdt(1,15,0)  OutputMin=[]  OutputMax=[]  ValidInPort=on  ReadyPort=off
      settings: SourceProductName=DSP System Toolbox  SourceProductBaseCode=DS
  Discrete FIR Filter HDL Optimized1 : dsphdlfiltering/Discrete FIR Filter HDL Optimized  Numerator=imag(Taps)  Sharing=off  SharingFactor=2  SimulateUsing=Code generation  roundingMode=Floor  overflowMode=off  CoefficientsDataTypeStr=Inherit: Same word length as input  CoefficientsMin=[]  CoefficientsMax=[]  OutputDataTypeStr=fixdt(1,15,0)  OutputMin=[]  OutputMax=[]  ValidInPort=on  ReadyPort=off
      settings: SourceProductName=DSP System Toolbox  SourceProductBaseCode=DS
  Logical Operator : Logic  AllPortsSameDT=off  OutDataTypeStr=boolean
  Out1 : Outport
  validOut : Outport  Port=2
  wires:
  In1/1 -> Discrete FIR Filter HDL Optimized1/1, Discrete FIR Filter HDL Optimized/1
  Discrete FIR Filter HDL Optimized/1 -> Add/1
  Add/1 -> Out1/1
  Logical Operator/1 -> validOut/1
  Discrete FIR Filter HDL Optimized/2 -> Logical Operator/1
  Discrete FIR Filter HDL Optimized1/2 -> Logical Operator/2
  Discrete FIR Filter HDL Optimized1/1 -> Add/2
  validIn/1 -> Discrete FIR Filter HDL Optimized1/2, Discrete FIR Filter HDL Optimized/2

== system Receiver/Receiver HDL/Frame Recover/Barker Locate/Measure Phase Ambiguity ==
  data : Inport  OutDataTypeStr=int16
  trigger : Inport  Port=2
  validIn : Inport  Port=3
  Find Max and Set Output Shift : Subsystem
  HDL Opt Complex FIR4 : Subsystem  mask{Taps=xPreambleSeq(end:-1:1).'}
  HDL Opt Complex FIR5 : Subsystem  mask{Taps=exp(-j*pi/2).*xPreambleSeq(end:-1:1).'}
  HDL Opt Complex FIR6 : Subsystem  mask{Taps=exp(-j*pi).*xPreambleSeq(end:-1:1).'}
  HDL Opt Complex FIR7 : Subsystem  mask{Taps=exp(-j*pi*3/2).*xPreambleSeq(end:-1:1).'}
  Logical Operator : Logic  Inputs=5  AllPortsSameDT=off  OutDataTypeStr=boolean
  PA : Outport  InitialOutput=0
  wires:
  data/1 -> HDL Opt Complex FIR4/1(In1), HDL Opt Complex FIR5/1(In1), HDL Opt Complex FIR7/1(In1), HDL Opt Complex FIR6/1(In1)
  HDL Opt Complex FIR4/1(Out1) -> Find Max and Set Output Shift/1(In1)
  HDL Opt Complex FIR5/1(Out1) -> Find Max and Set Output Shift/2(In2)
  HDL Opt Complex FIR6/1(Out1) -> Find Max and Set Output Shift/3(In4)
  HDL Opt Complex FIR7/1(Out1) -> Find Max and Set Output Shift/4(In5)
  Find Max and Set Output Shift/1(Out1) -> PA/1
  validIn/1 -> HDL Opt Complex FIR4/2(validIn), HDL Opt Complex FIR5/2(validIn), HDL Opt Complex FIR7/2(validIn), HDL Opt Complex FIR6/2(validIn)
  HDL Opt Complex FIR4/2(validOut) -> Logical Operator/1
  HDL Opt Complex FIR5/2(validOut) -> Logical Operator/2
  HDL Opt Complex FIR6/2(validOut) -> Logical Operator/3
  HDL Opt Complex FIR7/2(validOut) -> Logical Operator/4
  Logical Operator/1 -> Find Max and Set Output Shift/Enable
  trigger/1 -> Logical Operator/5

== system Receiver/Receiver HDL/Frame Recover/Equalization and Demodulation/2 Bit Descrambler ==
  note: This is a special Descrambler which can process 2 bits at a time
  u1 : Inport
  reset : Inport  Port=2
  Demux1 : Demux  Outputs=2
  MATLAB Function : MATLAB Function  TreatAsAtomicUnit=on
  Mux : Mux  Inputs=2
  Selector1 : Selector  IndexOptions=Index vector (dialog)  Indices=find(polynom(2:end))  OutputSizes=1
  Selector2 : Selector  IndexOptions=Index vector (dialog)  Indices=find(polynom(2:end))  OutputSizes=1
  input_xor1 : Logic  Operator=XOR  IconShape=distinctive  AllPortsSameDT=off  OutDataTypeStr=boolean
  input_xor2 : Logic  Operator=XOR  IconShape=distinctive  AllPortsSameDT=off  OutDataTypeStr=boolean
  state_xor1 : Logic  Operator=XOR  Inputs=1  IconShape=distinctive  AllPortsSameDT=off  OutDataTypeStr=boolean
  state_xor2 : Logic  Operator=XOR  Inputs=1  IconShape=distinctive  AllPortsSameDT=off  OutDataTypeStr=boolean
  y1 : Outport  InitialOutput=0
  wires:
  u1/1 -> Demux1/1, MATLAB Function/1(bits)
  reset/1 -> MATLAB Function/2(reset)
  MATLAB Function/1(bufferA) -> Selector1/1
  MATLAB Function/2(bufferB) -> Selector2/1
  Mux/1 -> y1/1
  state_xor1/1 -> input_xor1/1
  state_xor2/1 -> input_xor2/1
  input_xor2/1 -> Mux/2
  input_xor1/1 -> Mux/1
  Selector1/1 -> state_xor1/1
  Selector2/1 -> state_xor2/1
  Demux1/1 -> input_xor1/2
  Demux1/2 -> input_xor2/2  "data_in"

== system Receiver/Receiver HDL/Frame Recover/Equalization and Demodulation/DFE ==
  note: refTap=0 to disableEQ
  note: Generate training sequence when barker is found
  Trigger : Inport  PortDimensions=1
  data : Inport  Port=2  PortDimensions=1
      settings: SignalType=complex
  EQmu : Inport  Port=3
  DFE : Subsystem  mask{numFTaps=5, numBTaps=3, mu=0.01, refTap=2}
      mask prompts: numFTaps "Num Forward Taps"; numBTaps "Num Backward Taps"; mu "Step Size"; refTap "Reference Tap"
  Delay data so DFE can reset : Delay  DelayLength=1
  Delay ref so DFE can reset : Delay  DelayLength=1
  Equalizer : MATLAB Function  Commented=on  TreatAsAtomicUnit=on
  PN Sequence Generator : commseqgen3/PN Sequence Generator  poly='z^5 + z^3 + z^1 + 1'  ini_sta=[1 1 1 0 0]  outBitMaskSource=Dialog parameter  shift=0  outVarSiz=off  maxOutSizeMode=Dialog parameter  maxOutSize=[10 1]  Ts=-1  sampPerFrame=1  reset=on  bitPackedOutputs=on  outDataType=Smallest unsigned integer  numPackedBits=2  bitPackDataSigned=off  bitPackedOutDType=Smallest integer
      settings: SourceProductName=Communications System Toolbox
  Packeted To Unpacked : Subsystem
  QPSK Modulator Baseband : commdigbbndpm3/QPSK Modulator Baseband  InType=Bit  Enc=Binary  Ph=pi/4  outDtype=Fixed-point  outWordLen=16  outUDDataType=sfix(16)  outFracLenMode=User-defined  outFracLen=15  outDataTypeStr=fixdt(1,16,15)  outLastDataTypeStr=fixdt(1,16,15)
  Terminator1 : Terminator
  dataEQed : Outport
  start : Outport  Port=2
  wires:
  data/1 -> Delay data so DFE can reset/1
  PN Sequence Generator/1 -> Packeted To Unpacked/1(In1)
  Packeted To Unpacked/1(Out1) -> QPSK Modulator Baseband/1
  QPSK Modulator Baseband/1 -> Delay ref so DFE can reset/1
  DFE/3(start) -> start/1
  Trigger/1 -> DFE/1(reset), PN Sequence Generator/1
  DFE/2(err) -> Terminator1/1
  DFE/1(eqOut) -> dataEQed/1
  Delay data so DFE can reset/1 -> DFE/2(dataIn)
  Delay ref so DFE can reset/1 -> DFE/3(training)
  EQmu/1 -> DFE/4(EQmu)

== system Receiver/Receiver HDL/Frame Recover/Equalization and Demodulation/Subsystem ==
  <status> : Inport
  <s1> : Inport  Port=2
  <s2> : Inport  Port=3
  DEBUG: Header : MATLAB Function  TreatAsAtomicUnit=on
  wires:
  <s2>/1 -> DEBUG: Header/3(h2)
  <status>/1 -> DEBUG: Header/1(status)
  <s1>/1 -> DEBUG: Header/2(h1)

== system Receiver/Receiver HDL/Frame Recover/Frequency Recovery/Loop Filter ==
  note: Proportional-plus-Integrator Loop Filter,
      | Infinite DC Response to guarantee convergence
  e : Inport
  Add1 : Sum  RndMeth=Nearest  OutDataTypeStr=Inherit: Same as first input
  Add2 : Sum  OutDataTypeStr=Inherit: Same as first input
  Delay : Delay  DelayLength=1
  Delay3 : Delay  DelayLength=1
  Delay4 : Delay  DelayLength=1
  Gain : Gain  Gain=-1.0
  K1 : Gain  Gain=K2  OutDataTypeStr=Inherit: Same as input
  K2 : Gain  Gain=K1  OutDataTypeStr=Inherit: Same as input
  Sum2 : Sum  OutDataTypeStr=Inherit: Same as first input
  v : Outport
  wires:
  Gain/1 -> v/1
  Add2/1 -> Gain/1, Delay4/1
  Delay4/1 -> Add2/2
  Delay3/1 -> Add2/1
  Sum2/1 -> Delay3/1
  Delay/1 -> Add1/1
  K2/1 -> Add1/2, Delay/1
  e/1 -> K1/1, K2/1
  Add1/1 -> Sum2/2
  K1/1 -> Sum2/1

== system Receiver/Receiver HDL/Viterbi Decode/Buffer/DEBUG: Vitberi Check ==
  In1 : Inport
  In2 : Inport  Port=2
  In3 : Inport  Port=3
  In4 : Inport  Port=4
  Allow Viterbi Reset2 : Delay  DelayLength=1
  Allow Viterbi Reset3 : Delay  DelayLength=34
  Allow Viterbi Reset4 : Delay  DelayLength=1
  MATLAB Function2 : MATLAB Function  TreatAsAtomicUnit=on
  wires:
  Allow Viterbi Reset4/1 -> MATLAB Function2/2(enable)
  Allow Viterbi Reset3/1 -> MATLAB Function2/4(crc)
  In4/1 -> Allow Viterbi Reset3/1
  Allow Viterbi Reset2/1 -> MATLAB Function2/3(reset)
  In2/1 -> Allow Viterbi Reset4/1
  In1/1 -> MATLAB Function2/1(bits)
  In3/1 -> Allow Viterbi Reset2/1

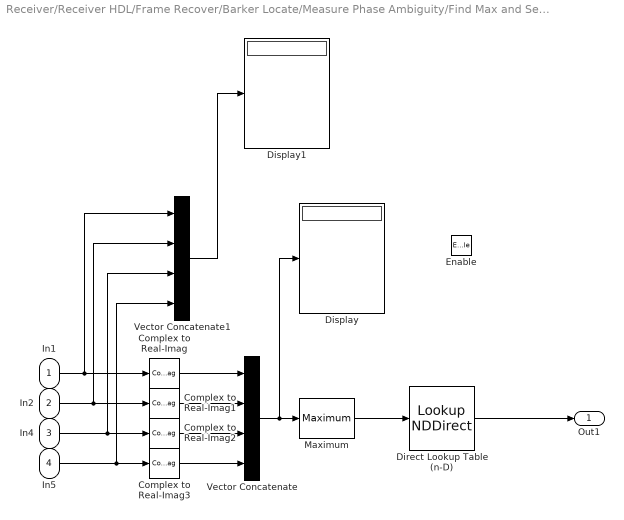
== system Receiver/Receiver HDL/Frame Recover/Barker Locate/Measure Phase Ambiguity/Find Max and Set Output Shift ==
  In1 : Inport
  In2 : Inport  Port=2
  In4 : Inport  Port=3
  In5 : Inport  Port=4
  Enable : EnablePort
  Complex to Real-Imag{,1..3} (4 alike) : ComplexToRealImag  Output=Imag
  Direct Lookup Table (n-D) : LookupNDDirect  NumberOfTableDimensions=1  Table=exp(-(0:pi/2:(pi*3/2)) .* 1i).'  DiagnosticForOutOfRangeInput=Error  TableDataTypeStr=fixdt(1,16,13)
  Display : Display
  Display1 : Display
  Maximum : dspstat3/Maximum  operation=maximum  fcn=Index  indexBase=Zero  operateOver=Each column  Dimension=1  InputProcessing=Columns as channels (frame based)  reset=None  roiEnable=off  roiType=Rectangles  roiPortion=Entire ROI  roiOutput=Individual statistics for each ROI  roiFlag=off  roundingMode=Floor  overflowMode=off  accumDataTypeStr=Inherit: Same as product output  accumLastDataTypeStr=Inherit: Same as product output
  Vector Concatenate : Concatenate  NumInputs=4
  Vector Concatenate1 : Concatenate  NumInputs=4
  Out1 : Outport  InitialOutput=0
  wires:
  Direct Lookup Table (n-D)/1 -> Out1/1
  In4/1 -> Vector Concatenate1/3, Complex to Real-Imag2/1
  In2/1 -> Vector Concatenate1/2, Complex to Real-Imag1/1
  In5/1 -> Vector Concatenate1/4, Complex to Real-Imag3/1
  In1/1 -> Vector Concatenate1/1, Complex to Real-Imag/1
  Maximum/1 -> Direct Lookup Table (n-D)/1
  Vector Concatenate/1 -> Display/1, Maximum/1
  Vector Concatenate1/1 -> Display1/1
  Complex to Real-Imag1/1 -> Vector Concatenate/2
  Complex to Real-Imag3/1 -> Vector Concatenate/4
  Complex to Real-Imag2/1 -> Vector Concatenate/3
  Complex to Real-Imag/1 -> Vector Concatenate/1

== system Receiver/Receiver HDL/Frame Recover/Barker Locate/Measure Phase Ambiguity/HDL Opt Complex FIR4 ==
  In1 : Inport
  validIn : Inport  Port=2
  Add : Sum  Inputs=+-  AccumDataTypeStr=fixdt(1,16,0)
  Complex to Real-Imag : ComplexToRealImag
  Discrete FIR Filter HDL Optimized : dsphdlfiltering/Discrete FIR Filter HDL Optimized  Numerator=real(Taps)  Sharing=off  SharingFactor=2  SimulateUsing=Code generation  roundingMode=Floor  overflowMode=off  CoefficientsDataTypeStr=Inherit: Same word length as input  CoefficientsMin=[]  CoefficientsMax=[]  OutputDataTypeStr=fixdt(1,16,0)  OutputMin=[]  OutputMax=[]  ValidInPort=on  ReadyPort=off
      settings: SourceProductName=DSP System Toolbox  SourceProductBaseCode=DS
  Discrete FIR Filter HDL Optimized1 : dsphdlfiltering/Discrete FIR Filter HDL Optimized  Numerator=imag(Taps)  Sharing=off  SharingFactor=2  SimulateUsing=Code generation  roundingMode=Floor  overflowMode=off  CoefficientsDataTypeStr=Inherit: Same word length as input  CoefficientsMin=[]  CoefficientsMax=[]  OutputDataTypeStr=fixdt(1,16,0)  OutputMin=[]  OutputMax=[]  ValidInPort=on  ReadyPort=off
      settings: SourceProductName=DSP System Toolbox  SourceProductBaseCode=DS
  Discrete FIR Filter HDL Optimized2 : dsphdlfiltering/Discrete FIR Filter HDL Optimized  Numerator=real(Taps)  Sharing=off  SharingFactor=2  SimulateUsing=Code generation  roundingMode=Floor  overflowMode=off  CoefficientsDataTypeStr=Inherit: Same word length as input  CoefficientsMin=[]  CoefficientsMax=[]  OutputDataTypeStr=fixdt(1,16,0)  OutputMin=[]  OutputMax=[]  ValidInPort=on  ReadyPort=off
      settings: SourceProductName=DSP System Toolbox  SourceProductBaseCode=DS
  Discrete FIR Filter HDL Optimized3 : dsphdlfiltering/Discrete FIR Filter HDL Optimized  Numerator=imag(Taps)  Sharing=off  SharingFactor=2  SimulateUsing=Code generation  roundingMode=Floor  overflowMode=off  CoefficientsDataTypeStr=Inherit: Same word length as input  CoefficientsMin=[]  CoefficientsMax=[]  OutputDataTypeStr=fixdt(1,16,0)  OutputMin=[]  OutputMax=[]  ValidInPort=on  ReadyPort=off
      settings: SourceProductName=DSP System Toolbox  SourceProductBaseCode=DS
  Logical Operator : Logic  Inputs=4  AllPortsSameDT=off  OutDataTypeStr=boolean
  Real-Imag to Complex : RealImagToComplex
  Subtract : Sum  OutDataTypeStr=int16
  Out1 : Outport
  validOut : Outport  Port=2
  wires:
  Discrete FIR Filter HDL Optimized/1 -> Add/1
  Logical Operator/1 -> validOut/1
  Discrete FIR Filter HDL Optimized/2 -> Logical Operator/1
  Discrete FIR Filter HDL Optimized1/2 -> Logical Operator/2
  Discrete FIR Filter HDL Optimized1/1 -> Add/2
  validIn/1 -> Discrete FIR Filter HDL Optimized3/2, Discrete FIR Filter HDL Optimized2/2, Discrete FIR Filter HDL Optimized1/2, Discrete FIR Filter HDL Optimized/2
  In1/1 -> Complex to Real-Imag/1
  Complex to Real-Imag/1 -> Discrete FIR Filter HDL Optimized3/1, Discrete FIR Filter HDL Optimized/1
  Discrete FIR Filter HDL Optimized2/2 -> Logical Operator/3
  Discrete FIR Filter HDL Optimized3/2 -> Logical Operator/4
  Complex to Real-Imag/2 -> Discrete FIR Filter HDL Optimized2/1, Discrete FIR Filter HDL Optimized1/1
  Discrete FIR Filter HDL Optimized2/1 -> Subtract/1
  Discrete FIR Filter HDL Optimized3/1 -> Subtract/2
  Real-Imag to Complex/1 -> Out1/1
  Subtract/1 -> Real-Imag to Complex/2
  Add/1 -> Real-Imag to Complex/1

== system Receiver/Receiver HDL/Frame Recover/Barker Locate/Measure Phase Ambiguity/HDL Opt Complex FIR5 ==
  In1 : Inport
  validIn : Inport  Port=2
  Add : Sum  Inputs=+-  AccumDataTypeStr=fixdt(1,16,0)
  Complex to Real-Imag : ComplexToRealImag
  Discrete FIR Filter HDL Optimized : dsphdlfiltering/Discrete FIR Filter HDL Optimized  Numerator=real(Taps)  Sharing=off  SharingFactor=2  SimulateUsing=Code generation  roundingMode=Floor  overflowMode=off  CoefficientsDataTypeStr=Inherit: Same word length as input  CoefficientsMin=[]  CoefficientsMax=[]  OutputDataTypeStr=fixdt(1,16,0)  OutputMin=[]  OutputMax=[]  ValidInPort=on  ReadyPort=off
      settings: SourceProductName=DSP System Toolbox  SourceProductBaseCode=DS
  Discrete FIR Filter HDL Optimized1 : dsphdlfiltering/Discrete FIR Filter HDL Optimized  Numerator=imag(Taps)  Sharing=off  SharingFactor=2  SimulateUsing=Code generation  roundingMode=Floor  overflowMode=off  CoefficientsDataTypeStr=Inherit: Same word length as input  CoefficientsMin=[]  CoefficientsMax=[]  OutputDataTypeStr=fixdt(1,16,0)  OutputMin=[]  OutputMax=[]  ValidInPort=on  ReadyPort=off
      settings: SourceProductName=DSP System Toolbox  SourceProductBaseCode=DS
  Discrete FIR Filter HDL Optimized2 : dsphdlfiltering/Discrete FIR Filter HDL Optimized  Numerator=real(Taps)  Sharing=off  SharingFactor=2  SimulateUsing=Code generation  roundingMode=Floor  overflowMode=off  CoefficientsDataTypeStr=Inherit: Same word length as input  CoefficientsMin=[]  CoefficientsMax=[]  OutputDataTypeStr=fixdt(1,16,0)  OutputMin=[]  OutputMax=[]  ValidInPort=on  ReadyPort=off
      settings: SourceProductName=DSP System Toolbox  SourceProductBaseCode=DS
  Discrete FIR Filter HDL Optimized3 : dsphdlfiltering/Discrete FIR Filter HDL Optimized  Numerator=imag(Taps)  Sharing=off  SharingFactor=2  SimulateUsing=Code generation  roundingMode=Floor  overflowMode=off  CoefficientsDataTypeStr=Inherit: Same word length as input  CoefficientsMin=[]  CoefficientsMax=[]  OutputDataTypeStr=fixdt(1,16,0)  OutputMin=[]  OutputMax=[]  ValidInPort=on  ReadyPort=off
      settings: SourceProductName=DSP System Toolbox  SourceProductBaseCode=DS
  Logical Operator : Logic  Inputs=4  AllPortsSameDT=off  OutDataTypeStr=boolean
  Real-Imag to Complex : RealImagToComplex
  Subtract : Sum  OutDataTypeStr=int16
  Out1 : Outport
  validOut : Outport  Port=2
  wires:
  Discrete FIR Filter HDL Optimized/1 -> Add/1
  Logical Operator/1 -> validOut/1
  Discrete FIR Filter HDL Optimized/2 -> Logical Operator/1
  Discrete FIR Filter HDL Optimized1/2 -> Logical Operator/2
  Discrete FIR Filter HDL Optimized1/1 -> Add/2
  validIn/1 -> Discrete FIR Filter HDL Optimized3/2, Discrete FIR Filter HDL Optimized2/2, Discrete FIR Filter HDL Optimized1/2, Discrete FIR Filter HDL Optimized/2
  In1/1 -> Complex to Real-Imag/1
  Complex to Real-Imag/1 -> Discrete FIR Filter HDL Optimized3/1, Discrete FIR Filter HDL Optimized/1
  Discrete FIR Filter HDL Optimized2/2 -> Logical Operator/3
  Discrete FIR Filter HDL Optimized3/2 -> Logical Operator/4
  Complex to Real-Imag/2 -> Discrete FIR Filter HDL Optimized2/1, Discrete FIR Filter HDL Optimized1/1
  Discrete FIR Filter HDL Optimized2/1 -> Subtract/1
  Discrete FIR Filter HDL Optimized3/1 -> Subtract/2
  Real-Imag to Complex/1 -> Out1/1
  Subtract/1 -> Real-Imag to Complex/2
  Add/1 -> Real-Imag to Complex/1

== system Receiver/Receiver HDL/Frame Recover/Barker Locate/Measure Phase Ambiguity/HDL Opt Complex FIR6 ==
  In1 : Inport
  validIn : Inport  Port=2
  Add : Sum  Inputs=+-  AccumDataTypeStr=fixdt(1,16,0)
  Complex to Real-Imag : ComplexToRealImag
  Discrete FIR Filter HDL Optimized : dsphdlfiltering/Discrete FIR Filter HDL Optimized  Numerator=real(Taps)  Sharing=off  SharingFactor=2  SimulateUsing=Code generation  roundingMode=Floor  overflowMode=off  CoefficientsDataTypeStr=Inherit: Same word length as input  CoefficientsMin=[]  CoefficientsMax=[]  OutputDataTypeStr=fixdt(1,16,0)  OutputMin=[]  OutputMax=[]  ValidInPort=on  ReadyPort=off
      settings: SourceProductName=DSP System Toolbox  SourceProductBaseCode=DS
  Discrete FIR Filter HDL Optimized1 : dsphdlfiltering/Discrete FIR Filter HDL Optimized  Numerator=imag(Taps)  Sharing=off  SharingFactor=2  SimulateUsing=Code generation  roundingMode=Floor  overflowMode=off  CoefficientsDataTypeStr=Inherit: Same word length as input  CoefficientsMin=[]  CoefficientsMax=[]  OutputDataTypeStr=fixdt(1,16,0)  OutputMin=[]  OutputMax=[]  ValidInPort=on  ReadyPort=off
      settings: SourceProductName=DSP System Toolbox  SourceProductBaseCode=DS
  Discrete FIR Filter HDL Optimized2 : dsphdlfiltering/Discrete FIR Filter HDL Optimized  Numerator=real(Taps)  Sharing=off  SharingFactor=2  SimulateUsing=Code generation  roundingMode=Floor  overflowMode=off  CoefficientsDataTypeStr=Inherit: Same word length as input  CoefficientsMin=[]  CoefficientsMax=[]  OutputDataTypeStr=fixdt(1,16,0)  OutputMin=[]  OutputMax=[]  ValidInPort=on  ReadyPort=off
      settings: SourceProductName=DSP System Toolbox  SourceProductBaseCode=DS
  Discrete FIR Filter HDL Optimized3 : dsphdlfiltering/Discrete FIR Filter HDL Optimized  Numerator=imag(Taps)  Sharing=off  SharingFactor=2  SimulateUsing=Code generation  roundingMode=Floor  overflowMode=off  CoefficientsDataTypeStr=Inherit: Same word length as input  CoefficientsMin=[]  CoefficientsMax=[]  OutputDataTypeStr=fixdt(1,16,0)  OutputMin=[]  OutputMax=[]  ValidInPort=on  ReadyPort=off
      settings: SourceProductName=DSP System Toolbox  SourceProductBaseCode=DS
  Logical Operator : Logic  Inputs=4  AllPortsSameDT=off  OutDataTypeStr=boolean
  Real-Imag to Complex : RealImagToComplex
  Subtract : Sum  OutDataTypeStr=int16
  Out1 : Outport
  validOut : Outport  Port=2
  wires:
  Discrete FIR Filter HDL Optimized/1 -> Add/1
  Logical Operator/1 -> validOut/1
  Discrete FIR Filter HDL Optimized/2 -> Logical Operator/1
  Discrete FIR Filter HDL Optimized1/2 -> Logical Operator/2
  Discrete FIR Filter HDL Optimized1/1 -> Add/2
  validIn/1 -> Discrete FIR Filter HDL Optimized3/2, Discrete FIR Filter HDL Optimized2/2, Discrete FIR Filter HDL Optimized1/2, Discrete FIR Filter HDL Optimized/2
  In1/1 -> Complex to Real-Imag/1
  Complex to Real-Imag/1 -> Discrete FIR Filter HDL Optimized3/1, Discrete FIR Filter HDL Optimized/1
  Discrete FIR Filter HDL Optimized2/2 -> Logical Operator/3
  Discrete FIR Filter HDL Optimized3/2 -> Logical Operator/4
  Complex to Real-Imag/2 -> Discrete FIR Filter HDL Optimized2/1, Discrete FIR Filter HDL Optimized1/1
  Discrete FIR Filter HDL Optimized2/1 -> Subtract/1
  Discrete FIR Filter HDL Optimized3/1 -> Subtract/2
  Real-Imag to Complex/1 -> Out1/1
  Subtract/1 -> Real-Imag to Complex/2
  Add/1 -> Real-Imag to Complex/1

== system Receiver/Receiver HDL/Frame Recover/Barker Locate/Measure Phase Ambiguity/HDL Opt Complex FIR7 ==
  In1 : Inport
  validIn : Inport  Port=2
  Add : Sum  Inputs=+-  AccumDataTypeStr=fixdt(1,16,0)
  Complex to Real-Imag : ComplexToRealImag
  Discrete FIR Filter HDL Optimized : dsphdlfiltering/Discrete FIR Filter HDL Optimized  Numerator=real(Taps)  Sharing=off  SharingFactor=2  SimulateUsing=Code generation  roundingMode=Floor  overflowMode=off  CoefficientsDataTypeStr=Inherit: Same word length as input  CoefficientsMin=[]  CoefficientsMax=[]  OutputDataTypeStr=fixdt(1,16,0)  OutputMin=[]  OutputMax=[]  ValidInPort=on  ReadyPort=off
      settings: SourceProductName=DSP System Toolbox  SourceProductBaseCode=DS
  Discrete FIR Filter HDL Optimized1 : dsphdlfiltering/Discrete FIR Filter HDL Optimized  Numerator=imag(Taps)  Sharing=off  SharingFactor=2  SimulateUsing=Code generation  roundingMode=Floor  overflowMode=off  CoefficientsDataTypeStr=Inherit: Same word length as input  CoefficientsMin=[]  CoefficientsMax=[]  OutputDataTypeStr=fixdt(1,16,0)  OutputMin=[]  OutputMax=[]  ValidInPort=on  ReadyPort=off
      settings: SourceProductName=DSP System Toolbox  SourceProductBaseCode=DS
  Discrete FIR Filter HDL Optimized2 : dsphdlfiltering/Discrete FIR Filter HDL Optimized  Numerator=real(Taps)  Sharing=off  SharingFactor=2  SimulateUsing=Code generation  roundingMode=Floor  overflowMode=off  CoefficientsDataTypeStr=Inherit: Same word length as input  CoefficientsMin=[]  CoefficientsMax=[]  OutputDataTypeStr=fixdt(1,16,0)  OutputMin=[]  OutputMax=[]  ValidInPort=on  ReadyPort=off
      settings: SourceProductName=DSP System Toolbox  SourceProductBaseCode=DS
  Discrete FIR Filter HDL Optimized3 : dsphdlfiltering/Discrete FIR Filter HDL Optimized  Numerator=imag(Taps)  Sharing=off  SharingFactor=2  SimulateUsing=Code generation  roundingMode=Floor  overflowMode=off  CoefficientsDataTypeStr=Inherit: Same word length as input  CoefficientsMin=[]  CoefficientsMax=[]  OutputDataTypeStr=fixdt(1,16,0)  OutputMin=[]  OutputMax=[]  ValidInPort=on  ReadyPort=off
      settings: SourceProductName=DSP System Toolbox  SourceProductBaseCode=DS
  Logical Operator : Logic  Inputs=4  AllPortsSameDT=off  OutDataTypeStr=boolean
  Real-Imag to Complex : RealImagToComplex
  Subtract : Sum  OutDataTypeStr=int16
  Out1 : Outport
  validOut : Outport  Port=2
  wires:
  Discrete FIR Filter HDL Optimized/1 -> Add/1
  Logical Operator/1 -> validOut/1
  Discrete FIR Filter HDL Optimized/2 -> Logical Operator/1
  Discrete FIR Filter HDL Optimized1/2 -> Logical Operator/2
  Discrete FIR Filter HDL Optimized1/1 -> Add/2
  validIn/1 -> Discrete FIR Filter HDL Optimized3/2, Discrete FIR Filter HDL Optimized2/2, Discrete FIR Filter HDL Optimized1/2, Discrete FIR Filter HDL Optimized/2
  In1/1 -> Complex to Real-Imag/1
  Complex to Real-Imag/1 -> Discrete FIR Filter HDL Optimized3/1, Discrete FIR Filter HDL Optimized/1
  Discrete FIR Filter HDL Optimized2/2 -> Logical Operator/3
  Discrete FIR Filter HDL Optimized3/2 -> Logical Operator/4
  Complex to Real-Imag/2 -> Discrete FIR Filter HDL Optimized2/1, Discrete FIR Filter HDL Optimized1/1
  Discrete FIR Filter HDL Optimized2/1 -> Subtract/1
  Discrete FIR Filter HDL Optimized3/1 -> Subtract/2
  Real-Imag to Complex/1 -> Out1/1
  Subtract/1 -> Real-Imag to Complex/2
  Add/1 -> Real-Imag to Complex/1
